simulink model "sliding_controller_rbdl"  (R2021a)
settings: Solver=FixedStepAuto  StartTime=0.0  StopTime=3  FixedStep=.01  RelTol=1e-3  EnableMultiTasking=on
model workspace (MAT data in the model file):
  SL_ROS_VariableLengthArrays_MaxSizes : object (value not decoded)
values from neighbouring files (symbols this model uses):
  alpha = [15  15]    [trying01.m]    (also in trying02.m = params(7,1).Value)
  beta = 0.25    [trying01.m]    (also in trying02.m = 0.25 + zeros(6,1))
  Bn0 = [Bn0_hip Bn0_knee Bn0_ankle Bn0_hip Bn0_knee Bn0_ankle ]    [trying01.m]    (also in trying02.m = params(1,1).Value)
  Bp0 = [Bp0_hip Bp0_knee Bp0_ankle Bp0_hip Bp0_knee Bp0_ankle ]    [trying01.m]    (also in trying02.m = params(2,1).Value)
  dampener = [0.30, 0; 0, 0.30]    [trying01.m]    (also in trying02.m = params(9,1).Value)
  delay = .00049    (= 0.00049)    [trying01.m]    (also in trying02.m)
  Dm1 = params.PD_const    [PD_start.m]    (also in trying01.m = [101.7013888888889 0 0 0 0 0; trying02.m = [101.7013888888889 0 0 0 0 0)
  exo_sat = 45    [trying01.m]    (also in trying02.m = 30)
  gamma = [15   15]    [trying01.m]
  human_sat = 20    [PD_start.m]    (also in trying01.m; trying02.m = 0)
  init_reorder = temp(init_order)    [trying01.m]    (also in trying02.m)
  interaction_sat = 6    [trying01.m]    (also in trying02.m)
  invMd = inv(Md)    [trying01.m]    (also in trying02.m)
  Km1 = [6120.116528948097 0 0 0 0 0 ... (first row only)    [trying01.m]    (also in trying02.m)
  Kn0 = [Kn0_hip Kn0_knee Kn0_ankle Kn0_hip Kn0_knee Kn0_ankle ]    [trying01.m]    (also in trying02.m = params(3,1).Value)
  Kp0 = [Kp0_hip Kp0_knee Kp0_ankle Kp0_hip Kp0_knee Kp0_ankle ]    [trying01.m]    (also in trying02.m = params(4,1).Value)
  lambda2 = [lambda_hip, 0, 0, 0, 0, 0 ... (first row only)    [trying01.m]    (also in trying02.m = params(8,1).Value)
  rho2 = [rho_hip, 0.0, 0.0, 0.0, 0.0, 0.0 ... (first row only)    [trying01.m]    (also in trying02.m = params(5,1).Value)
  spring = [0.30, 0; 0, 0.30]    [trying01.m]    (also in trying02.m = params(6,1).Value)
undefined symbols (not defined in the file or in its folder): Effort, l, mh, Position, Q, Qd, Qdd, Tau, Velocity
libraries: robotlib x20
(part 2 of 2)

== matlab function sliding_controller_rbdl/MATLAB Function5 ==
  data: u input; y output
function y = fcn(u)

reordered = [0 0 0 0 0 0 0]; 


% input: (-0.3642069399356842, 0.5383636355400085, 0.294272780418396, -0.31417930126190186, -5.772623990196735e-05, -0.5427972674369812, 0.0)
% 
% output: [-0.31417930126190186, 0.0, -0.3642069399356842, 0.5383636355400085, -5.772623990196735e-05, -0.5427972674369812, 0.2942727804u(3)18396]

reordered(1) = u(4);
reordered(2) = u(7);
reordered(3) = u(1);
reordered(4) = u(2);
reordered(5) = u(5);
reordered(6) = u(6);
reordered(7) = u(3);

y = reordered;

== matlab function sliding_controller_rbdl/Subsystem/MATLAB Function3 ==
  data: u input; y output
function y = fcn(u)

reordered = [0; 0; 0; 0; 0; 0]; 


% in: [-0.31417930126190186, 0.0, -0.3642069399356842, 0.5383636355400085, -5.772623990196735e-05, -0.5427972674369812, 0.294272780418396]


% out: (-0.3642069399356842, 0.5383636355400085, 0.294272780418396, -0.31417930126190186, -5.772623990196735e-05, -0.5427972674369812, 0.0)
% 





reordered(1) = u(3);
reordered(2) = u(4);
reordered(3) = u(7);
reordered(4) = u(1);
reordered(5) = u(5);
reordered(6) = u(6);


y = reordered;

== matlab function sliding_controller_rbdl/Subsystem/MATLAB Function4 ==
  data: u input; y output
function y = fcn(u)

reordered = [0; 0; 0; 0; 0; 0]; 


 

reordered(1) = u(2);
reordered(2) = u(3);
reordered(3) = u(4);
reordered(4) = u(1);
reordered(5) = u(5);
reordered(6) = u(6);



y = reordered;

== matlab function sliding_controller_rbdl/MATLAB Function - String Array Assign ==
  data: blankMsg input; msg output Bus: SL_Bus_sliding_controller_rbdl_RBDLInverseDynamicsReques_yqmb7i
function msg = stringArrayAssign(blankMsg)
% stringArrayAssign - Assign a string array in a ROS message
%
%  blankMsg (input): A bus for a 'sensor_msgs/JointState' message. This is 
%      used to initialize the output.
%  msg (output): A bus for a 'sensor_msgs/JointState' message message, with 
%      Name field set to a string array.
%
%   Copyright 2015 The MathWorks, Inc.

%#codegen

% Note: The datatype of 'msg' has been explicitly set to the appropriate 
% Simulink bus type ("SL_Bus_robotROSMessageUsageExample_sensor_msgs_JointState"). 
%
% If the model name is changed, the datatype needs to be changed as well:
%   1) Click "Edit Data" in the Editor toolstrip to open "Ports and Data Manager"
%   2) Select "msg". From the "Type" dropdown, select "--- Refresh data types ---"
%   3) Set datatype to "Bus: SL_Bus_<modelname>_sensor_msgs_JointState"

strArrayToAssign = {'exo'};
msg = blankMsg;
name = 'exo';
strLength = length(name);
% Set the number of strings in the string array.
% msg (sensor_msgs/JointState) includes the following fields
%           Name : array of std_msgs/String (string array)
%   Name_SL_Info : struct with fields CurrentLength, ReceivedLength
numStringsInArray = length(strArrayToAssign);
msg.ModelName_SL_Info.CurrentLength = uint32(strLength); % uint32(numStringsInArray);

msg.ModelName(1:strLength) = uint8(name);
msg.Q_SL_Info.CurrentLength = uint32(7);
msg.Qd_SL_Info.CurrentLength = uint32(7);
msg.Qdd_SL_Info.CurrentLength = uint32(7);

% % Set the individual strings in the array
% for idx=1:numStringsInArray
%     str = strArrayToAssign{idx};
%     strLength = length(str);
%     msg.ModelName(idx).Data(1:strLength) = uint8(str);
%     msg.Name(idx).Data_SL_Info.CurrentLength = uint32(strLength);
% end

== matlab function sliding_controller_rbdl/Controller/human controller/inv model 2/C ==
  data: m input; l input; q input; y output; qd input
function y = fcn(m, l, q, qd)



y = C(m, l, q, qd); % [m(2)*l(2)*qd(2)*qd(2)*sin(q(1)-q(2)); -m(2)*l(1)*qd(1)*qd(1)*sin(q(1)-q(2))];

== matlab function sliding_controller_rbdl/Controller/human controller/inv model 2/G ==
  data: m input; q input; y output
function y = fcn(m, q)
 y =  G(m,q);
end

== matlab function sliding_controller_rbdl/Controller/human controller/inv model 2/M ==
  data: m input; l input; q input; y output
function y = fcn(m, l, q)

y = M(m,l,q); % pinv([ (m(1)+m(2)) *l(1), m(2)*l(2)*cos(q(1)-q(2)); m(2)* l(1)*cos(q(1)-q(2)), m(2)*l(2)] );

end

== matlab function sliding_controller_rbdl/Subsystem/MATLAB Function1 ==
  data: u input; y output
function y = fcn(u)

reordered = [0; 0; 0; 0; 0; 0]; 


 

reordered(1) = u(2);
reordered(2) = u(3);
reordered(3) = u(4);
reordered(4) = u(1);
reordered(5) = u(5);
reordered(6) = u(6);



y = reordered;

== matlab function sliding_controller_rbdl/Controller/F->tau/Subsystem1/MATLAB Function ==
  data: q input; y output
function y = fcn(q)

l1 = 0.3240;
y = [-l1*sin(q(1)), 0; l1*cos(q(1)), 0 ];


end

== matlab function sliding_controller_rbdl/Subsystem/MATLAB Function2 ==
  data: u input; y output
function y = fcn(u)

reordered = [0; 0; 0; 0; 0; 0]; 


% in: [-0.31417930126190186, 0.0, -0.3642069399356842, 0.5383636355400085, -5.772623990196735e-05, -0.5427972674369812, 0.294272780418396]


% out: (-0.3642069399356842, 0.5383636355400085, 0.294272780418396, -0.31417930126190186, -5.772623990196735e-05, -0.5427972674369812, 0.0)
% 





reordered(1) = u(3);
reordered(2) = u(4);
reordered(3) = u(7);
reordered(4) = u(1);
reordered(5) = u(5);
reordered(6) = u(6);


y = reordered;

== matlab function sliding_controller_rbdl/Controller/F->tau/Subsystem1/MATLAB Function1 ==
  data: q input; y output
function y = fcn(q)

    l1 = 0.3240;
    l2 = 0.3900;
    y = [-l1*sin(q(1))-l2*sin(q(1)+q(2)), l1*cos(q(1)) + l2*sin(q(1)+q(2));...
         -l2*sin(q(1)+q(2)), l2*cos(q(1)+q(2))];
     
end

== matlab function sliding_controller_rbdl/Controller/ interaction sping-damper/human right ==
  data: q input; knee output; dknee output; qd input; ankle output; danke output
function [knee, dknee,ankle, danke]  = fcn(q, qd)


[knee, ankle, dknee, danke] = forward_kinimatics_leg(q,qd);
end
